simulink model "radiationForce_interp"  (R2022a)
settings: Solver=ode3  StartTime=0.0  StopTime=50  FixedStep=0.01  RelTol=1e-3
undefined symbols (not defined in the file): aRInterp, bRInterp, hydroCoeff, hydroVCoeff, tfRadAR_ROm, tfRadBR_ROm, tfRadCR_ROm, tfRadDR_ROm, w_WaveIndx
libraries: cstblocks x5, simulink x1
settings Model: Creator=tdemonte  LastModifiedBy=tdemonte

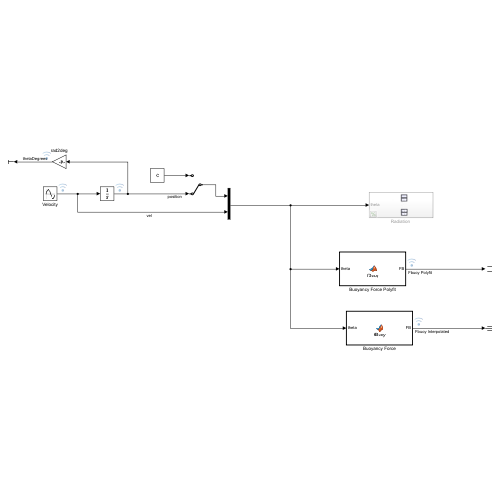
[thumbnail: Simulink's stored preview of the top-level diagram]
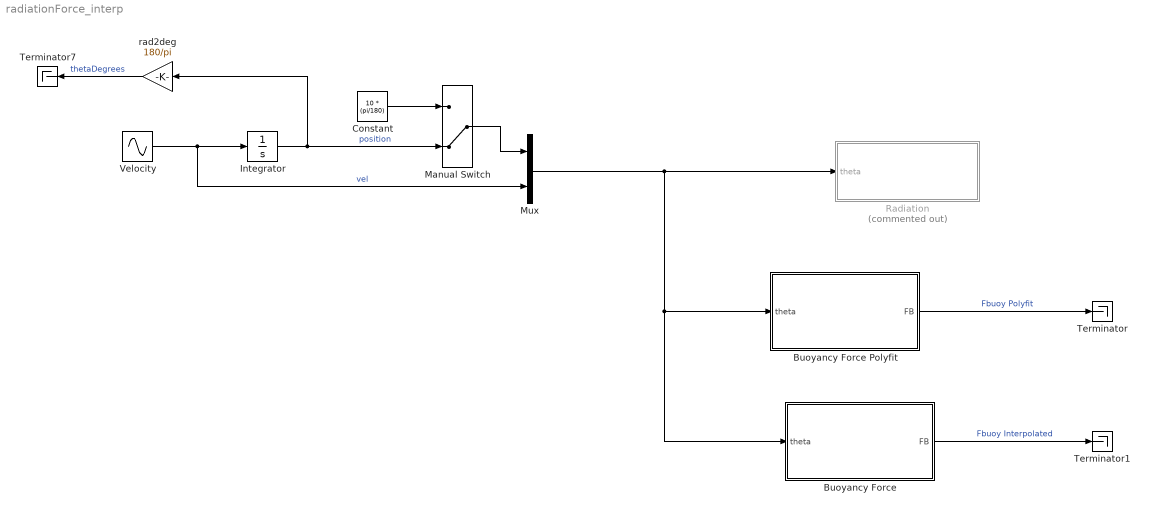
== system radiationForce_interp ==
  Buoyancy Force : MATLAB Function  TreatAsAtomicUnit=on
  Buoyancy Force Polyfit : MATLAB Function  TreatAsAtomicUnit=on
  Constant : Constant  Value=10 * (pi/180)
  Integrator : Integrator  InitialCondition=-1
  Manual Switch : ManualSwitch  CurrentSetting=0
  Mux : Mux  Inputs=2
  "Radiation " : Subsystem  Commented=on
  Terminator : Terminator
  Terminator1 : Terminator
  Terminator7 : Terminator
  Velocity : Sin  Amplitude=0.5  Frequency=0.5  SampleTime=0
  rad2deg : Gain  Gain=180/pi
  wires:
  Velocity/1 -> Mux/2, Integrator/1  "vel"
  Integrator/1 -> rad2deg/1, Manual Switch/2  "position"
  rad2deg/1 -> Terminator7/1  "thetaDegrees"
  Manual Switch/1 -> Mux/1
  Constant/1 -> Manual Switch/1
  Mux/1 -> Buoyancy Force/1(theta), Buoyancy Force Polyfit/1(theta), "Radiation "/1(theta)
  Buoyancy Force Polyfit/1(FB) -> Terminator/1  "Fbuoy Polyfit"
  Buoyancy Force/1(FB) -> Terminator1/1  "Fbuoy Interpolated"

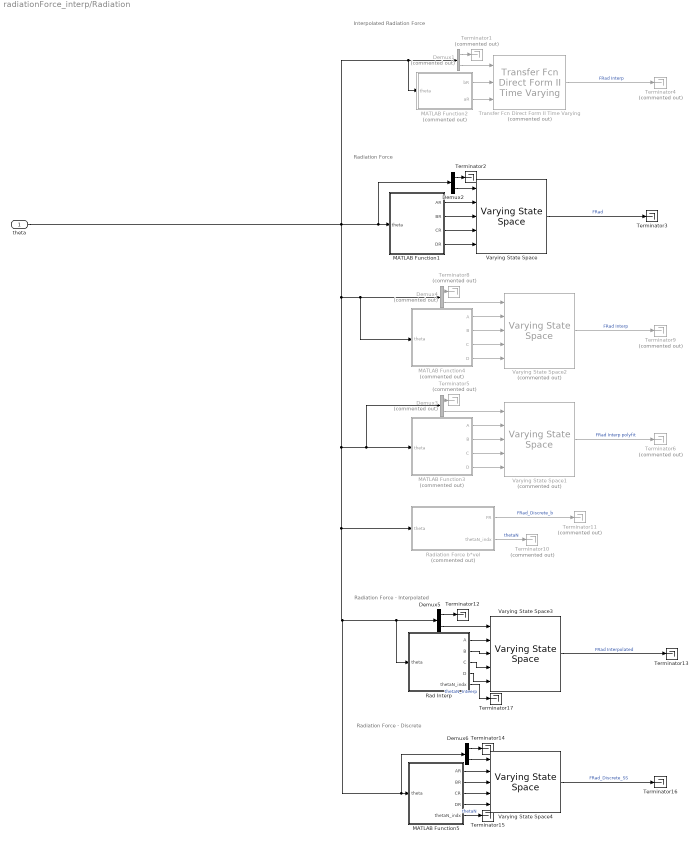
== system radiationForce_interp/Radiation  ==
  note: Radiation Force
  note: Interpolated Radiation Force
  note: Radiation Force - Interpolated
  note: Radiation Force - Discrete
  theta : Inport
  Demux1 : Demux  Commented=on  Outputs=2
  Demux2 : Demux  Outputs=2
  Demux3 : Demux  Commented=on  Outputs=2
  Demux4 : Demux  Commented=on  Outputs=2
  Demux5 : Demux  Outputs=2
  Demux6 : Demux  Outputs=2
  MATLAB Function1 : MATLAB Function  TreatAsAtomicUnit=on
  MATLAB Function2 : MATLAB Function  Commented=on  TreatAsAtomicUnit=on
  MATLAB Function3 : MATLAB Function  Commented=on  TreatAsAtomicUnit=on
  MATLAB Function4 : MATLAB Function  Commented=on  TreatAsAtomicUnit=on
  MATLAB Function5 : MATLAB Function  TreatAsAtomicUnit=on
  Rad Interp : MATLAB Function  TreatAsAtomicUnit=on
  Radiation Force b*vel : MATLAB Function  Commented=on  TreatAsAtomicUnit=on
  Terminator{1,4..6,8..11} (8 alike) : Terminator  Commented=on
  Terminator{2..3,12..17} (8 alike) : Terminator
  Transfer Fcn Direct Form II Time Varying : simulink/Additional Math & Discrete/Additional Discrete/Transfer Fcn Direct Form II Time Varying  Commented=on  vinit=0.0  DoSatur=off
      settings: SourceProductBaseCode=SL
  Varying State Space : cstblocks/Linear Parameter Varying/Varying State Space  x0=0  xNames=''  OutputX=off  OutputDX=off
  Varying State Space1 : cstblocks/Linear Parameter Varying/Varying State Space  Commented=on  x0=0  xNames=''  OutputX=off  OutputDX=off
  Varying State Space2 : cstblocks/Linear Parameter Varying/Varying State Space  Commented=on  x0=0  xNames=''  OutputX=off  OutputDX=off
  Varying State Space3 : cstblocks/Linear Parameter Varying/Varying State Space  x0=0  xNames=''  OutputX=off  OutputDX=off
  Varying State Space4 : cstblocks/Linear Parameter Varying/Varying State Space  x0=0  xNames=''  OutputX=off  OutputDX=off
  wires:
  Rad Interp/2(B) -> Varying State Space3/3
  Varying State Space/1 -> Terminator3/1  "FRad"
  Demux6/2 -> Varying State Space4/1
  theta/1 -> MATLAB Function2/1(theta), Demux1/1, Demux6/1, MATLAB Function5/1(theta), Rad Interp/1(theta), Demux5/1, Radiation Force b*vel/1(theta), MATLAB Function3/1(theta), Demux3/1, MATLAB Function4/1(theta), Demux4/1, Demux2/1, MATLAB Function1/1(theta)
  Demux2/2 -> Varying State Space/1
  MATLAB Function3/1(A) -> Varying State Space1/2
  MATLAB Function5/4(DR) -> Varying State Space4/5
  Rad Interp/4(D) -> Varying State Space3/5
  Varying State Space3/1 -> Terminator13/1  "FRad Interpolated"
  Demux3/1 -> Terminator5/1
  Varying State Space2/1 -> Terminator9/1  "FRad Interp"
  Radiation Force b*vel/1(FR) -> Terminator11/1  "FRad_Discrete_b"
  MATLAB Function5/3(CR) -> Varying State Space4/4
  MATLAB Function3/2(B) -> Varying State Space1/3
  MATLAB Function4/2(B) -> Varying State Space2/3
  Rad Interp/5(thetaN_indx) -> Terminator17/1  "thetaN_Inteerp"
  MATLAB Function3/4(D) -> Varying State Space1/5
  MATLAB Function3/3(C) -> Varying State Space1/4
  Varying State Space1/1 -> Terminator6/1  "FRad Interp polyfit"
  MATLAB Function1/2(BR) -> Varying State Space/3
  Demux4/1 -> Terminator8/1
  Demux5/1 -> Terminator12/1
  Rad Interp/3(C) -> Varying State Space3/4
  MATLAB Function2/2(aR) -> Transfer Fcn Direct Form II Time Varying/3
  Radiation Force b*vel/2(thetaN_indx) -> Terminator10/1  "thetaN"
  Varying State Space4/1 -> Terminator16/1  "FRad_Discrete_SS"
  Rad Interp/1(A) -> Varying State Space3/2
  Demux2/1 -> Terminator2/1
  MATLAB Function5/1(AR) -> Varying State Space4/2
  Demux3/2 -> Varying State Space1/1
  MATLAB Function4/4(D) -> Varying State Space2/5
  MATLAB Function4/1(A) -> Varying State Space2/2
  MATLAB Function1/3(CR) -> Varying State Space/4
  Demux4/2 -> Varying State Space2/1
  MATLAB Function4/3(C) -> Varying State Space2/4
  Demux5/2 -> Varying State Space3/1
  MATLAB Function5/5(thetaN_indx) -> Terminator15/1  "thetaN"
  Demux1/2 -> Transfer Fcn Direct Form II Time Varying/1
  Demux6/1 -> Terminator14/1
  MATLAB Function5/2(BR) -> Varying State Space4/3
  Transfer Fcn Direct Form II Time Varying/1 -> Terminator4/1  "FRad Interp"
  MATLAB Function1/4(DR) -> Varying State Space/5
  Demux1/1 -> Terminator1/1
  MATLAB Function2/1(bR) -> Transfer Fcn Direct Form II Time Varying/2
  MATLAB Function1/1(AR) -> Varying State Space/2

== matlab function radiationForce_interp/Radiation /MATLAB Function5 ==
  data: theta input; AR output size=[6 6]; BR output size=[6 1]; CR output size=[1 6]; DR output size=1; hydroCoeff parameter; tfRadAR_ROm parameter; tfRadBR_ROm parameter; tfRadCR_ROm parameter; tfRadDR_ROm parameter; thetaN_indx output size=1
function [AR, BR, CR, DR, thetaN_indx] = RadTFCoeffs(theta,hydroCoeff, tfRadAR_ROm, tfRadBR_ROm, tfRadCR_ROm, tfRadDR_ROm)
% This function extracts the coefficients of the Radiation Transfer
% Function based on discrete thetas. 

% Inputs: 
% theta0      = current states condition
% hydrovCoeff = time-variable hydrodynamic coefficients
% thetaN      = pitch angle index

% Outputs: 
% bR    = radiation force (N) 

theta1 = theta(1); 
% Find the index for the discretized theta 
theta1N = wrapToPi(theta1); 

if abs(rad2deg(theta1N)) >= 95 
    theta1N = pi - abs(theta1N);
end 

 
thetaN = find(deg2rad(hydroCoeff.theta) > abs(theta1N),1); 

% % Get transfer function coefficients depending on the discretized angle. 
AR       = zeros(6,6); 
BR       = zeros(6,1); 
CR       = zeros(1,6); 
DR       = 0; 

thetaN_indx = 0; 
thetaN_indx = thetaN(1);

AR(:,:)       = tfRadAR_ROm(:,(thetaN_indx-1)*6+1:(thetaN_indx*6)); % A Matrix Coefficients

BR(:,1)       = tfRadBR_ROm(:,thetaN_indx); % A Matrix Coefficients
CR(1,:)       = tfRadCR_ROm(1,(thetaN_indx-1)*6+1:(thetaN_indx*6)); % A Matrix Coefficients
DR(1)         = tfRadDR_ROm(thetaN_indx); % A Matrix Coefficients

== matlab function radiationForce_interp/Radiation /Radiation Force b*vel ==
  data: theta input size=[1 2]; FR output double size=1; hydroCoeff parameter; hydroVCoeff parameter; w_WaveIndx parameter; thetaN_indx output
function [FR, thetaN_indx] = fRad(theta,hydroCoeff, hydroVCoeff,w_WaveIndx)

% States: 
theta1  = theta(1); % (1) theta:  pitch angle response
theta2  = theta(2); % (2) thetaD: pitch angle velocity

% Find the index for the discretized theta 

theta1N = wrapToPi(theta1); 

if abs(rad2deg(theta1N)) >= 95 
    theta1N = pi - abs(theta1N);
end 


thetaN = find(deg2rad(hydroCoeff.theta) > abs(theta1N),1); 

thetaN_indx = 0; 
thetaN_indx = thetaN(1);

b  = hydroVCoeff.KR(w_WaveIndx,thetaN); % Radiation Damping Coefficient  

FR = 0; 
FR(1) = b*theta2; % Buoyancy Force for Time-Varying Hydrodynamics (N)

== matlab function radiationForce_interp/Radiation /MATLAB Function3 ==
  data: theta input; A output size=[6 6]; B output size=[6 1]; hydroVCoeff parameter; C output size=[1 6]; D output size=1
function [A,B,C,D] = RadTFCoeffs(theta, hydroVCoeff)
% This function extracts the coefficients of the Radiation Transfer
% Function based on previously fitted data between discretized thetas. 

% Inputs: 
% theta0      = current states condition
% hydrovCoeff = time-variable hydrodynamic coefficients
% thetaN      = pitch angle index

% Outputs: 
% bR    = numerator 
% aR    = denominator 

% States: 
theta1  = theta(1); % (1) theta:  pitch angle response
% theta2  = theta(2); % (2) thetaD: pitch angle velocity

theta1 = wrapToPi(theta1); 
theta1D = rad2deg(theta1); 
% Find the index for the discretized theta 
if abs(theta1D) >= 95
    theta1D = 180 - abs(theta1D);
end 

% % Get transfer function coefficients depending on the discretized angle. 
aR       = zeros(1,7); 
bR       = zeros(1,7);

aR(1)    = 1; % But no lead denominator
aR(2)    = polyval(hydroVCoeff.aRFit(2,:), theta1D,[], hydroVCoeff.aR_mu(2,:));
aR(3)    = polyval(hydroVCoeff.aRFit(3,:), theta1D,[], hydroVCoeff.aR_mu(3,:));
aR(4)    = polyval(hydroVCoeff.aRFit(4,:), theta1D,[], hydroVCoeff.aR_mu(4,:));
aR(5)    = polyval(hydroVCoeff.aRFit(5,:), theta1D,[], hydroVCoeff.aR_mu(5,:));
aR(6)    = polyval(hydroVCoeff.aRFit(6,:), theta1D,[], hydroVCoeff.aR_mu(6,:));
aR(7)    = polyval(hydroVCoeff.aRFit(7,:), theta1D,[], hydroVCoeff.aR_mu(7,:));

bR(1)    = polyval(hydroVCoeff.bRFit(1,:), theta1D,[], hydroVCoeff.bR_mu(1,:));
bR(2)    = polyval(hydroVCoeff.bRFit(2,:), theta1D,[], hydroVCoeff.bR_mu(2,:));
bR(3)    = polyval(hydroVCoeff.bRFit(3,:), theta1D,[], hydroVCoeff.bR_mu(3,:));
bR(4)    = polyval(hydroVCoeff.bRFit(4,:), theta1D,[], hydroVCoeff.bR_mu(4,:));
bR(5)    = polyval(hydroVCoeff.bRFit(5,:), theta1D,[], hydroVCoeff.bR_mu(5,:));
bR(6)    = polyval(hydroVCoeff.bRFit(6,:), theta1D,[], hydroVCoeff.bR_mu(6,:));
bR(7)    = polyval(hydroVCoeff.bRFit(7,:), theta1D,[], hydroVCoeff.bR_mu(7,:));

% % Get transfer function coefficients depending on the discretized angle. 
A       = zeros(6,6); 
B       = zeros(6,1); 
C       = zeros(1,6); 
D       = 0; 

[A(:,:), B(:,1), C(1,:), D(1)] = tf2ss(bR,aR);

== matlab function radiationForce_interp/Radiation /MATLAB Function4 ==
  data: theta input; A output size=[6 6]; B output size=[6 1]; hydroCoeff parameter; C output size=[1 6]; D output size=1; aRInterp parameter; bRInterp parameter
function [A,B,C,D] = RadTFCoeffs(theta, hydroCoeff, aRInterp, bRInterp)
% This function extracts the coefficients of the Radiation Transfer
% Function based on previously fitted data between discretized thetas. 

% Inputs: 
% theta0      = current states condition
% hydrovCoeff = time-variable hydrodynamic coefficients
% thetaN      = pitch angle index

% Outputs: 
% bR    = numerator 
% aR    = denominator 

% States: 
theta1  = theta(1); % (1) theta:  pitch angle response
% theta2  = theta(2); % (2) thetaD: pitch angle velocity


% Find the index for the discretized theta 
theta1N = wrapToPi(theta1); 

if abs(rad2deg(theta1N)) >= 95 
    theta1N = pi - abs(theta1N); 
end 

thetaN = find(deg2rad(hydroCoeff.fineTheta) > abs(theta1N),1)-1; 
% % Get transfer function coefficients depending on the discretized angle. 
aR       = zeros(1,7); 
bR       = zeros(1,7);

aR(1,:)    = aRInterp(:,thetaN);
bR(1,:)    = bRInterp(:,thetaN);

% % Get transfer function coefficients depending on the discretized angle. 
A       = zeros(6,6); 
B       = zeros(6,1); 
C       = zeros(1,6); 
D       = 0; 

[A(:,:), B(:,1), C(1,:), D(1)] = tf2ss(bR,aR);

== matlab function radiationForce_interp/Radiation /MATLAB Function2 ==
  data: theta input; bR output size=[1 7]; aR output size=[1 6]; hydroVCoeff parameter
function [bR, aR] = RadTFCoeffs(theta, hydroVCoeff)
% This function extracts the coefficients of the Radiation Transfer
% Function based on previously fitted data between discretized thetas. 

% Inputs: 
% theta0      = current states condition
% hydrovCoeff = time-variable hydrodynamic coefficients
% thetaN      = pitch angle index

% Outputs: 
% bR    = numerator 
% aR    = denominator 

% States: 
theta1  = theta(1); % (1) theta:  pitch angle response
% theta2  = theta(2); % (2) thetaD: pitch angle velocity

theta1 = wrapToPi(theta1); 
theta1D = rad2deg(theta1); 
% Find the index for the discretized theta 
if abs(theta1D) >= 95
    theta1D = 180 - abs(theta1D);
end 

% % Get transfer function coefficients depending on the discretized angle. 
aR       = zeros(1,6); 
bR       = zeros(1,7);

aR(1)    = 1; % But no lead denominator
aR(1)    = polyval(hydroVCoeff.aRFit(2,:), theta1D,[], hydroVCoeff.aR_mu(2,:));
aR(2)    = polyval(hydroVCoeff.aRFit(3,:), theta1D,[], hydroVCoeff.aR_mu(3,:));
aR(3)    = polyval(hydroVCoeff.aRFit(4,:), theta1D,[], hydroVCoeff.aR_mu(4,:));
aR(4)    = polyval(hydroVCoeff.aRFit(5,:), theta1D,[], hydroVCoeff.aR_mu(5,:));
aR(5)    = polyval(hydroVCoeff.aRFit(6,:), theta1D,[], hydroVCoeff.aR_mu(6,:));
aR(6)    = polyval(hydroVCoeff.aRFit(7,:), theta1D,[], hydroVCoeff.aR_mu(7,:));

bR(1)    = polyval(hydroVCoeff.bRFit(1,:), theta1D,[], hydroVCoeff.bR_mu(1,:));
bR(2)    = polyval(hydroVCoeff.bRFit(2,:), theta1D,[], hydroVCoeff.bR_mu(2,:));
bR(3)    = polyval(hydroVCoeff.bRFit(3,:), theta1D,[], hydroVCoeff.bR_mu(3,:));
bR(4)    = polyval(hydroVCoeff.bRFit(4,:), theta1D,[], hydroVCoeff.bR_mu(4,:));
bR(5)    = polyval(hydroVCoeff.bRFit(5,:), theta1D,[], hydroVCoeff.bR_mu(5,:));
bR(6)    = polyval(hydroVCoeff.bRFit(6,:), theta1D,[], hydroVCoeff.bR_mu(6,:));
bR(7)    = polyval(hydroVCoeff.bRFit(7,:), theta1D,[], hydroVCoeff.bR_mu(7,:));

== matlab function radiationForce_interp/Buoyancy Force ==
  data: theta input size=[1 2]; FB output double size=1; hydroCoeff parameter; hydroVCoeff parameter
function FB = fBuoy(theta,hydroCoeff, hydroVCoeff)

% States: 
theta1  = theta(1); % (1) theta:  pitch angle response
% theta2  = theta(2); % (2) thetaD: pitch angle velocity

% Find the index for the discretized theta 
theta1N = wrapToPi(theta1); 

if abs(rad2deg(theta1N)) >= 95 
    theta1N = pi - abs(theta1N);
end 

thetaN = find(deg2rad(hydroCoeff.fineTheta) > abs(theta1N),1); 


%% Interpolation
c  = hydroVCoeff.cInterp(thetaN); % Hydrostatic restoring coefficient. (t) 
FB = 0; 
FB(1) = c*theta1; % Buoyancy Force for Time-Varying Hydrodynamics (N)

== matlab function radiationForce_interp/Radiation /Rad Interp ==
  data: theta input; A output size=[6 6]; B output size=[6 1]; hydroCoeff parameter; C output size=[1 6]; D output size=1; aRInterp parameter; bRInterp parameter; thetaN_indx output size=1
function [A,B,C,D,thetaN_indx] = RadTFCoeffs(theta, hydroCoeff, aRInterp, bRInterp)
% This function extracts the coefficients of the Radiation Transfer
% Function based on previously fitted data between discretized thetas. 

% Inputs: 
% theta0      = current states condition
% hydrovCoeff = time-variable hydrodynamic coefficients
% thetaN      = pitch angle index

% Outputs: 
% bR    = numerator 
% aR    = denominator 

% States: 
theta1  = theta(1); % (1) theta:  pitch angle response
% theta2  = theta(2); % (2) thetaD: pitch angle velocity


% Find the index for the discretized theta 
theta1N = wrapToPi(theta1); 

if abs(rad2deg(theta1N)) >= 95
    theta1N = pi - abs(theta1N); 
end 

thetaN = find(deg2rad(hydroCoeff.fineTheta) > abs(theta1N),1); 
thetaN_indx = 0; 
thetaN_indx = thetaN(1);

% % Get transfer function coefficients depending on the discretized angle. 
aR       = zeros(1,7); 
bR       = zeros(1,7);

aR(1,:)    = aRInterp(:,thetaN);
bR(1,:)    = bRInterp(:,thetaN);


% % Get transfer function coefficients depending on the discretized angle. 
A       = zeros(6,6); 
B       = zeros(6,1); 
C       = zeros(1,6); 
D       = 0; 

[A(:,:), B(:,1), C(1,:), D(1)] = tf2ss(bR,aR);

== matlab function radiationForce_interp/Buoyancy Force Polyfit ==
  data: theta input size=[1 2]; FB output double size=1; hydroVCoeff parameter
function FB = fBuoy(theta, hydroVCoeff)

% States: 
theta1  = theta(1); % (1) theta:  pitch angle response
% theta2  = theta(2); % (2) thetaD: pitch angle velocity

theta1 = wrapToPi(theta1); 
theta1D = rad2deg(theta1); 
% Find the index for the discretized theta 
if abs(theta1D) >= 95
    theta1D = 180 - abs(theta1D);
end 

c  = zeros(1,1); 
c  = polyval(hydroVCoeff.cFit, abs(theta1D),[], hydroVCoeff.c_mu); % Hydrostatic restoring coefficient. (t) 

FB    = 0; 
FB(1) = c*theta1; % Buoyancy Force for Time-Varying Hydrodynamics (N)

== matlab function radiationForce_interp/Radiation /MATLAB Function1 ==
  data: theta input; AR output size=[6 6]; BR output size=[6 1]; CR output size=[1 6]; DR output size=1; hydroCoeff parameter; tfRadAR_ROm parameter; tfRadBR_ROm parameter; tfRadCR_ROm parameter; tfRadDR_ROm parameter
function [AR, BR, CR, DR] = RadTFCoeffs(theta,hydroCoeff, tfRadAR_ROm, tfRadBR_ROm, tfRadCR_ROm, tfRadDR_ROm)
% This function extracts the coefficients of the Radiation Transfer
% Function based on previously fitted data between discretized thetas. 

% Inputs: 
% theta0      = current states condition
% hydrovCoeff = time-variable hydrodynamic coefficients
% thetaN      = pitch angle index

% Outputs: 
% bR    = radiation force (N) 

theta1 = theta(1); 
% Find the index for the discretized theta 
theta1N = wrapToPi(theta1); 

if abs(rad2deg(theta1N)) >= 95 
    theta1N = pi - abs(theta1N);
end 


thetaN = find(deg2rad(hydroCoeff.theta) > abs(theta1N),1); 

% % Get transfer function coefficients depending on the discretized angle. 
AR       = zeros(6,6); 
BR       = zeros(6,1); 
CR       = zeros(1,6); 
DR       = 0; 

thetaN_indx = thetaN(1);


AR(:,:)       = tfRadAR_ROm(:,(thetaN_indx-1)*6+1:(thetaN_indx*6)); % A Matrix Coefficients

BR(:,1)       = tfRadBR_ROm(:,thetaN_indx); % A Matrix Coefficients
CR(1,:)       = tfRadCR_ROm(1,(thetaN_indx-1)*6+1:(thetaN_indx*6)); % A Matrix Coefficients
DR(1)         = tfRadDR_ROm(thetaN_indx); % A Matrix Coefficients
